simulink model "untitled"  (R2016b)
settings: Solver=VariableStepAuto  StartTime=0.0  StopTime=10.0  RelTol=1e-3
settings Model: Creator=ivan_  LastModifiedBy=ivan_

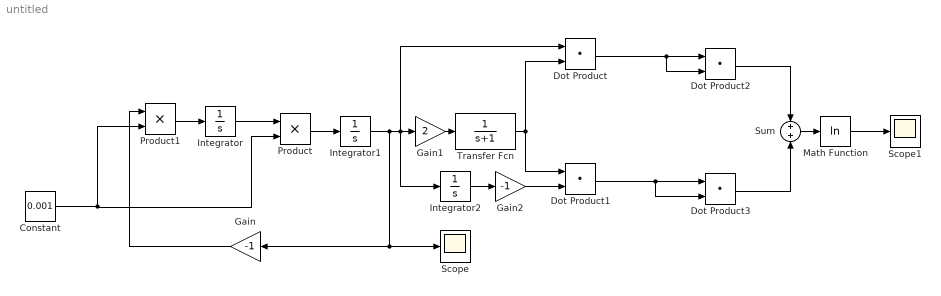
== system untitled ==
  Constant : Constant  Value=0.001
  Dot Product{,1..3} (4 alike) : DotProduct  InputSameDT=on  OutDataTypeStr=Inherit: Inherit via internal rule
  Gain : Gain  Gain=-1
  Gain1 : Gain  Gain=2
  Gain2 : Gain  Gain=-1
  Integrator : Integrator  InitialCondition=1
  Integrator1 : Integrator
  Integrator2 : Integrator  InitialCondition=-1
  Math Function : Math  Operator=log  SaturateOnIntegerOverflow=on
  Product : Product
  Product1 : Product
  Scope : Scope
  Scope1 : Scope
  Sum : Sum  Inputs=+|+
  Transfer Fcn : TransferFcn  Denominator=[1 1]
  wires:
  Integrator/1 -> Product/1
  Product/1 -> Integrator1/1
  Product1/1 -> Integrator/1
  Constant/1 -> Product/2, Product1/2
  Integrator1/1 -> Integrator2/1, Dot Product/1, Gain1/1, Scope/1, Gain/1
  Gain/1 -> Product1/1
  Transfer Fcn/1 -> Dot Product/2, Dot Product1/1
  Gain1/1 -> Transfer Fcn/1
  Integrator2/1 -> Gain2/1
  Gain2/1 -> Dot Product1/2
  Dot Product1/1 -> Dot Product3/2, Dot Product3/1
  Dot Product/1 -> Dot Product2/2, Dot Product2/1
  Dot Product3/1 -> Sum/2
  Dot Product2/1 -> Sum/1
  Sum/1 -> Math Function/1
  Math Function/1 -> Scope1/1
